simulink model "phev"  (Simulink 8.1)
settings: Solver=ode3  StartTime=0.0  StopTime=6*3600  FixedStep=1  RelTol=1e-3
undefined symbols (not defined in the file): range
libraries: simulink x4
settings Model: Creator=sfrank1  LastModifiedBy=sfrank1
settings DataIOCC: SignalLoggingSaveFormat=Dataset
settings OptimizationCC: ExpressionDepthLimit=128
settings DebuggingCC: FcnCallInpInsideContextMsg=EnableAllAsError
settings GRTTargetCC: CombineOutputUpdateFcns=on  GRTInterface=off

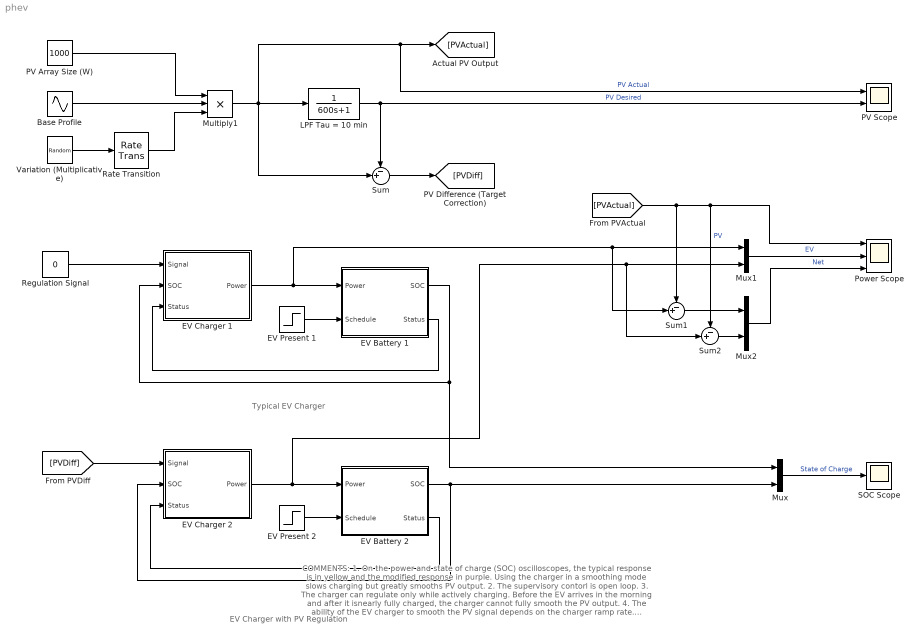
== system phev ==
  note: COMMENTS:
      | 1. On the power and state of charge (SOC) oscilloscopes, the typical
      | response is in yellow and the modified response in purple. Using
      | the charger in a smoothing mode slows charging but greatly smooths
      | PV output.
      | 2. The supervisory contorl is open loop.
      | 3. The charger can regulate only while actively charging. Before the
      | EV arrives in the morning and after it isnearly fully charged, the
      | charger cannot fully smooth the PV output.
      | 4. The ability of the EV charger to smooth the PV signal depends on
      | the charger ramp rate. Reducing the ramp rate allows rapid PV
      | fluctuations to "bleed through" into the net power consumption.
      | (Try a maximum ramp rate of 400 W/s, for instance.)
  note: Typical EV Charger
  note: EV Charger with
      | PV Regulation
  Base Profile : Sin  Frequency=(2*pi)/(12*3600)  SampleTime=0
  EV Battery 1 : Subsystem  mask(Electric Vehicle Battery){capacity=24000, initSOC=0.4}
      mask prompts: capacity "Battery capacity (Wh)"; initSOC "Initial state of charge (fraction)"
  EV Battery 2 : Subsystem  mask(Electric Vehicle Battery){capacity=24000, initSOC=0.4}
      mask prompts: capacity "Battery capacity (Wh)"; initSOC "Initial state of charge (fraction)"
  EV Charger 1 : Subsystem  mask{rating=6240, capacity=24000, maxresponse=0, ramp=1000}
      mask prompts: rating "Charger rating (W)"; capacity "Connected EV battery capacity (Wh)"; maxresponse "Desired response capability (W)"; ramp "Maximum ramp rate (W/s)"
  EV Charger 2 : Subsystem  mask{rating=6240, capacity=24000, maxresponse=1000, ramp=1000}
      mask prompts: rating "Charger rating (W)"; capacity "Connected EV battery capacity (Wh)"; maxresponse "Desired response capability (W)"; ramp "Maximum ramp rate (W/s)"
  EV Present 1 : Step  Time=3600  SampleTime=0
  EV Present 2 : Step  Time=3600  SampleTime=0
  LPF Tau = 10 min : TransferFcn  Denominator=[600 1]
  Multiply1 : Product  Inputs=***
  Mux : Mux  Inputs=2
  Mux1 : Mux  Inputs=2
  Mux2 : Mux  Inputs=2
  PV Array Size (W) : Constant  Value=1000
  PV Scope : Scope  NumInputPorts=2
      settings: TimeRange=25000  YMin=0~0  YMax=1500~800  SaveName=ScopeData3
  Power Scope : Scope  NumInputPorts=3
      settings: TimeRange=25000  YMin=0~0~-5000  YMax=1500~8000~10000
  Rate Transition : RateTransition
  Regulation Signal : Constant  Value=0
  SOC Scope : Scope
      settings: TimeRange=25000  YMin=0  YMax=1
  Sum : Sum  Inputs=-+|
  Sum1 : Sum  Inputs=-+|
  Sum2 : Sum  Inputs=-+|
  Variation (Multiplicative) : UniformRandomNumber  Minimum=0.1  Maximum=1.1  Seed=42  SampleTime=10
  wires:
  Variation (Multiplicative)/1 -> Rate Transition/1
  EV Charger 1/1(Power) -> Sum1/2, Mux1/1, EV Battery 1/1(Power)
  Base Profile/1 -> Multiply1/2
  PV Array Size (W)/1 -> Multiply1/1
  Rate Transition/1 -> Multiply1/3
  LPF Tau = 10 min/1 -> PV Scope/2, Sum/1  "PV Desired"
  Multiply1/1 -> Sum/2, LPF Tau = 10 min/1, PV Scope/1, [PVActual]  "PV Actual"
  Sum/1 -> [PVDiff]
  EV Present 1/1 -> EV Battery 1/2(Schedule)
  Regulation Signal/1 -> EV Charger 1/1(Signal)
  EV Battery 1/1(SOC) -> Mux/1, EV Charger 1/2(SOC)
  EV Battery 1/2(Status) -> EV Charger 1/3(Status)
  EV Charger 2/1(Power) -> Sum2/2, Mux1/2, EV Battery 2/1(Power)
  EV Present 2/1 -> EV Battery 2/2(Schedule)
  EV Battery 2/1(SOC) -> EV Charger 2/2(SOC), Mux/2
  EV Battery 2/2(Status) -> EV Charger 2/3(Status)
  [PVDiff] -> EV Charger 2/1(Signal)
  Mux/1 -> SOC Scope/1  "State of Charge"
  [PVActual] -> Sum1/1, Sum2/1, Power Scope/1  "PV"
  Mux1/1 -> Power Scope/2  "EV"
  Sum1/1 -> Mux2/1
  Sum2/1 -> Mux2/2
  Mux2/1 -> Power Scope/3  "Net"

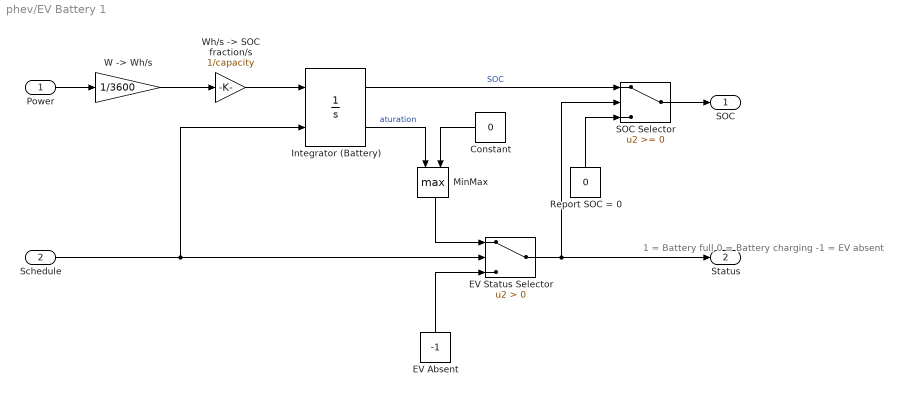
== system phev/EV Battery 1 ==
  note: 1 = Battery full
      | 0 = Battery charging
      | -1 = EV absent
  Power : Inport
  Schedule : Inport  Port=2
  Constant : Constant  Value=0
  EV Absent : Constant  Value=-1
  EV Status Selector : Switch  Criteria=u2 > Threshold
  Integrator (Battery) : Integrator  ExternalReset=rising  InitialCondition=initSOC  LimitOutput=on  UpperSaturationLimit=1  LowerSaturationLimit=0  ShowSaturationPort=on  ContinuousStateAttributes='SOC'
  MinMax : MinMax  Function=max  Inputs=2
  Report SOC = 0 : Constant  Value=0
  SOC Selector : Switch
  "W -> Wh/s" : Gain  Gain=1/3600
  "Wh/s -> SOC fraction/s" : Gain  Gain=1/capacity
  SOC : Outport
  Status : Outport  Port=2
  wires:
  "W -> Wh/s"/1 -> "Wh/s -> SOC fraction/s"/1
  Power/1 -> "W -> Wh/s"/1
  "Wh/s -> SOC fraction/s"/1 -> Integrator (Battery)/1
  Schedule/1 -> EV Status Selector/2, Integrator (Battery)/2
  EV Absent/1 -> EV Status Selector/3
  EV Status Selector/1 -> SOC Selector/2, Status/1
  Integrator (Battery)/2 -> MinMax/1  "aturation"
  MinMax/1 -> EV Status Selector/1
  Constant/1 -> MinMax/2
  Integrator (Battery)/1 -> SOC Selector/1  "SOC"
  SOC Selector/1 -> SOC/1
  Report SOC = 0/1 -> SOC Selector/3

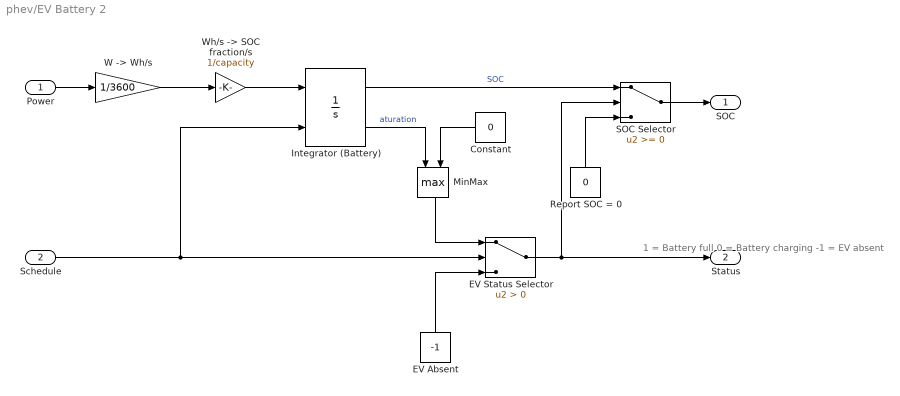
== system phev/EV Battery 2 ==
  note: 1 = Battery full
      | 0 = Battery charging
      | -1 = EV absent
  Power : Inport
  Schedule : Inport  Port=2
  Constant : Constant  Value=0
  EV Absent : Constant  Value=-1
  EV Status Selector : Switch  Criteria=u2 > Threshold
  Integrator (Battery) : Integrator  ExternalReset=rising  InitialCondition=initSOC  LimitOutput=on  UpperSaturationLimit=1  LowerSaturationLimit=0  ShowSaturationPort=on  ContinuousStateAttributes='SOC'
  MinMax : MinMax  Function=max  Inputs=2
  Report SOC = 0 : Constant  Value=0
  SOC Selector : Switch
  "W -> Wh/s" : Gain  Gain=1/3600
  "Wh/s -> SOC fraction/s" : Gain  Gain=1/capacity
  SOC : Outport
  Status : Outport  Port=2
  wires:
  "W -> Wh/s"/1 -> "Wh/s -> SOC fraction/s"/1
  Power/1 -> "W -> Wh/s"/1
  "Wh/s -> SOC fraction/s"/1 -> Integrator (Battery)/1
  Schedule/1 -> EV Status Selector/2, Integrator (Battery)/2
  EV Absent/1 -> EV Status Selector/3
  EV Status Selector/1 -> SOC Selector/2, Status/1
  Integrator (Battery)/2 -> MinMax/1  "aturation"
  MinMax/1 -> EV Status Selector/1
  Constant/1 -> MinMax/2
  Integrator (Battery)/1 -> SOC Selector/1  "SOC"
  SOC Selector/1 -> SOC/1
  Report SOC = 0/1 -> SOC Selector/3

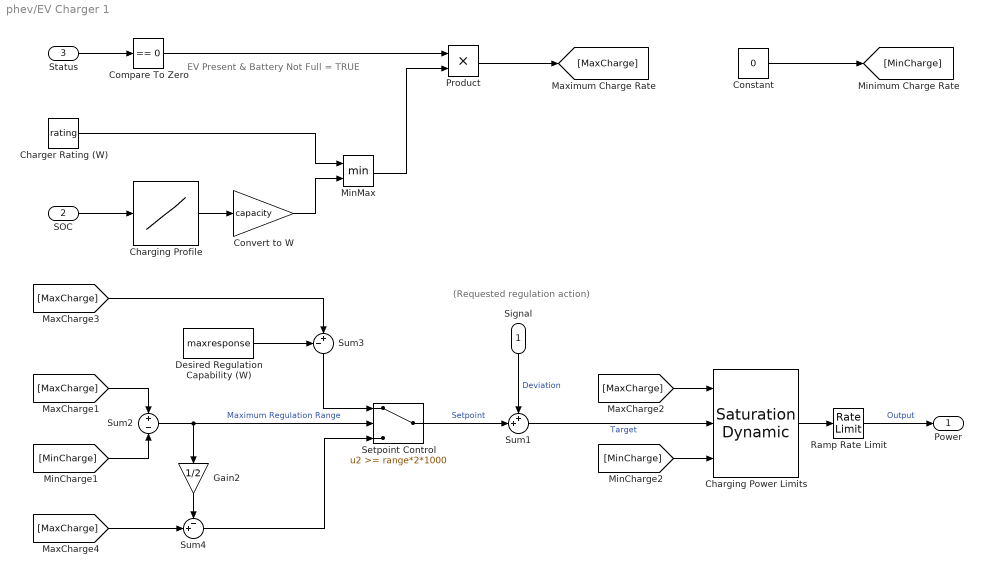
== system phev/EV Charger 1 ==
  note: EV Present & Battery Not Full = TRUE
  note: (Requested regulation action)
  Signal : Inport
  SOC : Inport  Port=2
  Status : Inport  Port=3
  Charger Rating (W) : Constant  Value=rating
  Charging Power Limits : simulink/Discontinuities/Saturation Dynamic  OutMin=[]  OutMax=[]  OutDataTypeStr=Inherit: Same as second input  OutDataType=fixdt(1, 16)  OutScaling=2^-10  DoSatur=off
  Charging Profile : Lookup_n-D  NumberOfTableDimensions=1  BreakpointsForDimension1=[0.00 0.10 0.20 0.80 0.99 1.00]  IndexSearchMethod=Linear search  BeginIndexSearchUsingPreviousIndexResult=on  Table=[0.10 0.20 1.00 1.00 0.02 0.00]  ExtrapMethod=Clip  UseLastTableValue=on  RndMeth=Simplest  InputSameDT=on
  Compare To Zero : simulink/Logic and Bit Operations/Compare To Zero  relop===  OutDataTypeStr=boolean
  Constant : Constant  Value=0
  Convert to W : Gain  Gain=capacity
  Desired Regulation Capability (W) : Constant  Value=maxresponse
  Gain2 : Gain  Gain=1/2
  MinMax : MinMax  Inputs=2
  Product : Product
  Ramp Rate Limit : RateLimiter  RisingSlewLimit=ramp  FallingSlewLimit=-ramp  SampleTimeMode=inherited
  Setpoint Control : Switch  Threshold=range*2*1000
  Sum1 : Sum  Inputs=++|
  Sum2 : Sum  Inputs=+-
  Sum3 : Sum  Inputs=-+|
  Sum4 : Sum  Inputs=-+|
  Power : Outport
  wires:
  Sum1/1 -> Charging Power Limits/2  "Target"
  Ramp Rate Limit/1 -> Power/1  "Output"
  SOC/1 -> Charging Profile/1
  Charging Profile/1 -> Convert to W/1
  Charging Power Limits/1 -> Ramp Rate Limit/1
  Status/1 -> Compare To Zero/1
  Compare To Zero/1 -> Product/1
  Convert to W/1 -> MinMax/2
  Charger Rating (W)/1 -> MinMax/1
  MinMax/1 -> Product/2
  Product/1 -> [MaxCharge]
  Constant/1 -> [MinCharge]
  Signal/1 -> Sum1/1  "Deviation"
  [MaxCharge] -> Charging Power Limits/1
  [MinCharge] -> Charging Power Limits/3
  Sum2/1 -> Gain2/1, Setpoint Control/2  "Maximum Regulation Range"
  [MaxCharge] -> Sum2/1
  [MinCharge] -> Sum2/2
  Setpoint Control/1 -> Sum1/2  "Setpoint"
  Sum3/1 -> Setpoint Control/1
  [MaxCharge] -> Sum4/2
  Gain2/1 -> Sum4/1
  Sum4/1 -> Setpoint Control/3
  [MaxCharge] -> Sum3/2
  Desired Regulation Capability (W)/1 -> Sum3/1

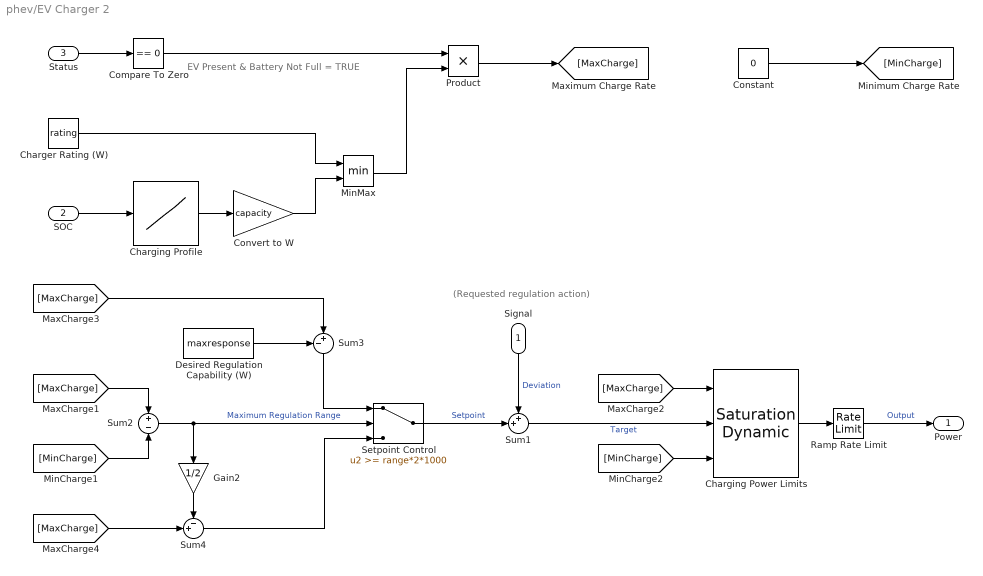
== system phev/EV Charger 2 ==
  note: (Requested regulation action)
  note: EV Present & Battery Not Full = TRUE
  Signal : Inport
  SOC : Inport  Port=2
  Status : Inport  Port=3
  Charger Rating (W) : Constant  Value=rating
  Charging Power Limits : simulink/Discontinuities/Saturation Dynamic  OutMin=[]  OutMax=[]  OutDataTypeStr=Inherit: Same as second input  OutDataType=fixdt(1, 16)  OutScaling=2^-10  DoSatur=off
  Charging Profile : Lookup_n-D  NumberOfTableDimensions=1  BreakpointsForDimension1=[0.00 0.10 0.20 0.80 0.99 1.00]  IndexSearchMethod=Linear search  BeginIndexSearchUsingPreviousIndexResult=on  Table=[0.10 0.20 1.00 1.00 0.02 0.00]  ExtrapMethod=Clip  UseLastTableValue=on  RndMeth=Simplest  InputSameDT=on
  Compare To Zero : simulink/Logic and Bit Operations/Compare To Zero  relop===  OutDataTypeStr=boolean
  Constant : Constant  Value=0
  Convert to W : Gain  Gain=capacity
  Desired Regulation Capability (W) : Constant  Value=maxresponse
  Gain2 : Gain  Gain=1/2
  MinMax : MinMax  Inputs=2
  Product : Product
  Ramp Rate Limit : RateLimiter  RisingSlewLimit=ramp  FallingSlewLimit=-ramp  SampleTimeMode=inherited
  Setpoint Control : Switch  Threshold=range*2*1000
  Sum1 : Sum  Inputs=++|
  Sum2 : Sum  Inputs=+-
  Sum3 : Sum  Inputs=-+|
  Sum4 : Sum  Inputs=-+|
  Power : Outport
  wires:
  Desired Regulation Capability (W)/1 -> Sum3/1
  [MaxCharge] -> Sum3/2
  Sum4/1 -> Setpoint Control/3
  Gain2/1 -> Sum4/1
  [MaxCharge] -> Sum4/2
  Sum3/1 -> Setpoint Control/1
  Setpoint Control/1 -> Sum1/2  "Setpoint"
  [MinCharge] -> Sum2/2
  [MaxCharge] -> Sum2/1
  Sum2/1 -> Setpoint Control/2, Gain2/1  "Maximum Regulation Range"
  [MinCharge] -> Charging Power Limits/3
  [MaxCharge] -> Charging Power Limits/1
  Signal/1 -> Sum1/1  "Deviation"
  Constant/1 -> [MinCharge]
  Product/1 -> [MaxCharge]
  MinMax/1 -> Product/2
  Charger Rating (W)/1 -> MinMax/1
  Convert to W/1 -> MinMax/2
  Compare To Zero/1 -> Product/1
  Status/1 -> Compare To Zero/1
  Charging Power Limits/1 -> Ramp Rate Limit/1
  Charging Profile/1 -> Convert to W/1
  SOC/1 -> Charging Profile/1
  Ramp Rate Limit/1 -> Power/1  "Output"
  Sum1/1 -> Charging Power Limits/2  "Target"
